simulink model "ar2_pos_123"  (R2019b)
settings: Solver=VariableStepAuto  StartTime=0.0  StopTime=10
libraries: simulink x3
settings Model: Creator=ah501846  LastModifiedBy=ah501846

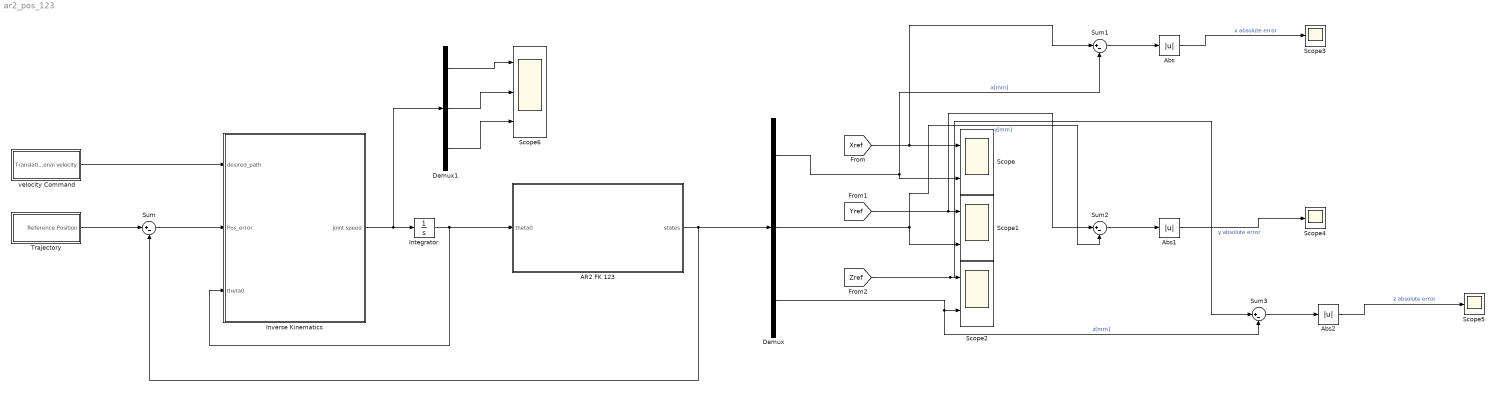
== system ar2_pos_123 ==
  AR2 FK 123 : MATLAB Function  TreatAsAtomicUnit=on
  Abs : Abs
  Abs1 : Abs
  Abs2 : Abs
  Demux : Demux  Outputs=3
  Demux1 : Demux  Outputs=3
  Integrator : Integrator  InitialCondition=[40 50 130 ]'*pi/180
  Inverse Kinematics : Subsystem
  Scope : Scope  NumInputPorts=2
  Scope1 : Scope  NumInputPorts=2
  Scope2 : Scope  NumInputPorts=2
  Scope3 : Scope
  Scope4 : Scope
  Scope5 : Scope
  Scope6 : Scope  NumInputPorts=3
  Sum{,1..3} (4 alike) : Sum  Inputs=|+-
  "Trajectory " : Subsystem
  velocity Command : Subsystem
  wires:
  "Trajectory "/1(Reference Position) -> Sum/1
  Sum/1 -> Inverse Kinematics/2(Pos_error)
  Inverse Kinematics/1(joint speed) -> Demux1/1, Integrator/1
  velocity Command/1(Translational velocity) -> Inverse Kinematics/1(desired_path)
  Integrator/1 -> AR2 FK 123/1(theta0), Inverse Kinematics/3(theta0)
  AR2 FK 123/1(states) -> Sum/2, Demux/1
  Abs1/1 -> Scope4/1  "y absolute error"
  Sum2/1 -> Abs1/1
  [Zref] -> Sum3/1, Scope2/1
  Sum1/1 -> Abs/1
  Abs/1 -> Scope3/1  "x absolute error"
  Demux/2 -> Scope1/2, Sum2/2  "y[mm]"
  Demux/3 -> Sum3/2, Scope2/2  "z[mm]"
  [Yref] -> Sum2/1, Scope1/1
  [Xref] -> Sum1/1, Scope/1
  Demux/1 -> Scope/2, Sum1/2  "x[mm]"
  Abs2/1 -> Scope5/1  "z absolute error"
  Sum3/1 -> Abs2/1
  Demux1/3 -> Scope6/3
  Demux1/2 -> Scope6/2
  Demux1/1 -> Scope6/1

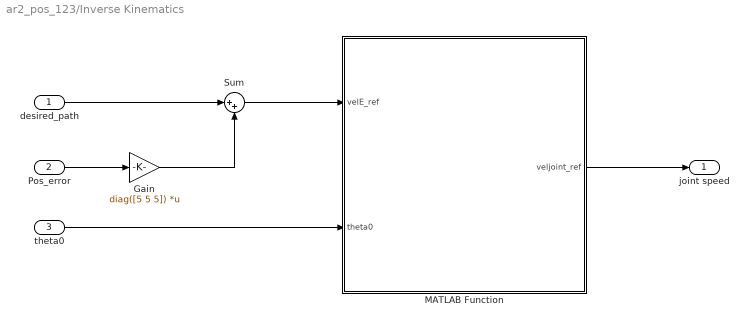
== system ar2_pos_123/Inverse Kinematics ==
  desired_path : Inport
  Pos_error : Inport  Port=2
  theta0 : Inport  Port=3
  Gain : Gain  Gain=diag([5 5 5])  Multiplication=Matrix(K*u)
  MATLAB Function : MATLAB Function  TreatAsAtomicUnit=on
  Sum : Sum  Inputs=|++
  joint speed : Outport  VectorParamsAs1DForOutWhenUnconnected=off
  wires:
  MATLAB Function/1(veljoint_ref) -> joint speed/1
  theta0/1 -> MATLAB Function/2(theta0)
  desired_path/1 -> Sum/1
  Sum/1 -> MATLAB Function/1(velE_ref)
  Pos_error/1 -> Gain/1
  Gain/1 -> Sum/2

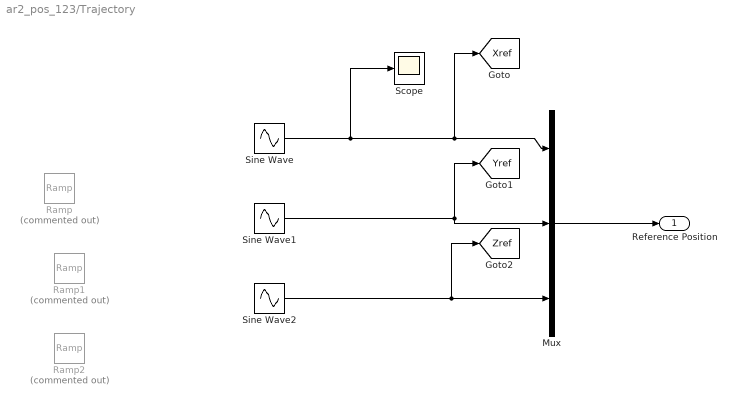
== system ar2_pos_123/Trajectory  ==
  Mux : Mux  Inputs=3
  Ramp : simulink/Sources/Ramp  Commented=on  slope=1  start=0  InitialOutput=195
  Ramp1 : simulink/Sources/Ramp  Commented=on  slope=1  start=0  InitialOutput=165
  Ramp2 : simulink/Sources/Ramp  Commented=on  slope=1  start=0  InitialOutput=-52
  Scope : Scope
  Sine Wave : Sin  Amplitude=50  Bias=195  SampleTime=0
  Sine Wave1 : Sin  Amplitude=50  Bias=165  SampleTime=0
  Sine Wave2 : Sin  Amplitude=50  Bias=-52  SampleTime=0
  Reference Position : Outport  VectorParamsAs1DForOutWhenUnconnected=off
  tag scope: Xref=global, Yref=global, Zref=global
  wires:
  Mux/1 -> Reference Position/1
  Sine Wave/1 -> Scope/1, Mux/1, [Xref]
  Sine Wave1/1 -> [Yref], Mux/2
  Sine Wave2/1 -> Mux/3, [Zref]

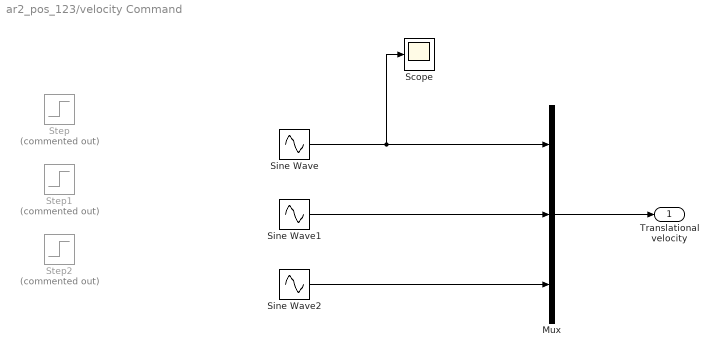
== system ar2_pos_123/velocity Command ==
  Mux : Mux  Inputs=3
  Scope : Scope
  Sine Wave : Sin  Amplitude=50  Phase=pi/2  SampleTime=0
  Sine Wave1 : Sin  Amplitude=50  Phase=pi/2  SampleTime=0
  Sine Wave2 : Sin  Amplitude=50  Phase=pi/2  SampleTime=0
  Step : Step  Commented=on  Time=10  SampleTime=0
  Step1 : Step  Commented=on  Time=10  SampleTime=0
  Step2 : Step  Commented=on  Time=10  SampleTime=0
  Translational velocity : Outport  VectorParamsAs1DForOutWhenUnconnected=off
  wires:
  Mux/1 -> Translational velocity/1
  Sine Wave/1 -> Scope/1, Mux/1
  Sine Wave1/1 -> Mux/2
  Sine Wave2/1 -> Mux/3

== matlab function ar2_pos_123/AR2 FK 123 ==
  data: states output; theta0 input
% function to calculate analytical Jacobian 
function states = manipFK(theta0)
%% Inputs
theta1 = theta0(1);
theta2 = theta0(2);
theta3 = theta0(3);
%% DH parameters
d1 = 169.77;    a1 = 64.2;  alpha1 = -90*pi/180;    
d2 = 0;         a2 = 305;   alpha2 = 0;             
d3 = 0;         a3 = 0;     alpha3 = 90*pi/180;     
d4 = -222.63;   a4 = 0;     alpha4 = -90*pi/180;    
d5 = 0;         a5 = 0;     alpha5 = 90*pi/180;     
d6 = -36.25;    a6 = 0;     alpha6 = 0;             
%% Direct Forward Kinematics
DH1 = [cos(theta1) -sin(theta1)*cos(alpha1) sin(theta1)*sin(alpha1) a1*cos(theta1);
       sin(theta1) cos(theta1)*cos(alpha1) -cos(theta1)*sin(alpha1) a1*sin(theta1); 
        0           sin(alpha1)             cos(alpha1)             d1;
        0 0 0 1];
DH2 = [cos(theta2) -sin(theta2)*cos(alpha2) sin(theta2)*sin(alpha2)     a2*cos(theta2);
        sin(theta2) cos(theta2)*cos(alpha2) -cos(theta2)*sin(alpha2)    a2*sin(theta2);
        0           sin(alpha2)             cos(alpha2)                 d2;
    0 0 0 1];
DH3 = [cos(theta3) -sin(theta3)*cos(alpha3) sin(theta3)*sin(alpha3) a3*cos(theta3);
    sin(theta3) cos(theta3)*cos(alpha3) -cos(theta3)*sin(alpha3)    a3*sin(theta3);
    0 sin(alpha3) cos(alpha3)                                       d3;
    0 0 0 1];
%% Homogeneous Transformation Matrix of the end effector to the base
HT3 = DH1*DH2*DH3;
%% Position
l1 = d1;
l2 = a2;
l3 = d4;
x = cos(theta1)*(l2*cos(theta2) + l3*sin(theta2+theta3));
y = sin(theta1) * (l2*cos(theta2) + l3*sin(theta2+theta3) );
z = l1 - l3*cos(theta2 + theta3) + l2*sin(theta2);
%% Outputs
states =  [x y z]';

== matlab function ar2_pos_123/Inverse Kinematics/MATLAB Function ==
  data: velE_ref input; veljoint_ref output; theta0 input
function veljoint_ref = trajectoryIK(velE_ref,theta0)

d1 = 169.77;    a1 = 64.2;  alpha1 = -90*pi/180;
d2 = 0;         a2 = 305;   alpha2 = 0;
d3 = 0;         a3 = 0;     alpha3 = 90*pi/180;
d4 = -222.63;   a4 = 0;     alpha4 = -90*pi/180;
d5 = 0;         a5 = 0;     alpha5 = 90*pi/180;
d6 = -36.25;    a6 = 0;     alpha6 = 0;

theta1 = theta0(1);
theta2 = theta0(2);
theta3 = theta0(3);
theta23 = theta2 + theta3;

cth1 = cos(theta1);
cth2 = cos(theta2);
cth3 = cos(theta3);
cth23 = cos(theta23);
sth1 = sin(theta1);
sth2 = sin(theta2);
sth3 = sin(theta3);
sth23 = sin(theta23);

cal1 = cos(alpha1);
cal2 = cos(alpha2);
cal3 = cos(alpha3);

sal1 = sin(alpha1);
sal2 = sin(alpha2);
sal3 = sin(alpha3);


% Jv3 = ([[d3*(cal2*sal1*cth1 - sal2*sth1*sth2 + cal1*sal2*cth1*cth2) - a1*sth1 + d2*sal1*cth1 + a3*sth3*(sal1*sal2*cth1 + cal2*sth1*sth2 - cal1*cal2*cth1*cth2) - a2*cth2*sth1 - a3*cth3*(cth2*sth1 + cal1*cth1*sth2) - a2*cal1*cth1*sth2, d3*(sal2*cth1*cth2 - cal1*sal2*sth1*sth2) - a2*cth1*sth2 - a3*sth3*(cal2*cth1*cth2 - cal1*cal2*sth1*sth2) - a3*cth3*(cth1*sth2 + cal1*cth2*sth1) - a2*cal1*cth2*sth1, - a3*sth3*(cth1*cth2 - cal1*sth1*sth2) - a3*cth3*(cal2*cth1*sth2 - sal1*sal2*sth1 + cal1*cal2*cth2*sth1)]; 
% [a1*cth1 + d3*(cal2*sal1*sth1 + sal2*cth1*sth2 + cal1*sal2*cth2*sth1) + a2*cth1*cth2 + d2*sal1*sth1 - a3*sth3*(cal2*cth1*sth2 - sal1*sal2*sth1 + cal1*cal2*cth2*sth1) + a3*cth3*(cth1*cth2 - cal1*sth1*sth2) - a2*cal1*sth1*sth2, d3*(sal2*cth2*sth1 + cal1*sal2*cth1*sth2) - a2*sth1*sth2 - a3*sth3*(cal2*cth2*sth1 + cal1*cal2*cth1*sth2) - a3*cth3*(sth1*sth2 - cal1*cth1*cth2) + a2*cal1*cth1*cth2, - a3*sth3*(cth2*sth1 + cal1*cth1*sth2) - a3*cth3*(sal1*sal2*cth1 + cal2*sth1*sth2 - cal1*cal2*cth1*cth2)]; 
% [0, a2*sal1*cth2 + a3*sal1*cth2*cth3 + d3*sal1*sal2*sth2 - a3*cal2*sal1*sth2*sth3, a3*cth3*(cal1*sal2 + cal2*sal1*cth2) - a3*sal1*sth2*sth3]]); 


l1 = d1;
l2 = a2;
l3 = d4;

Jv3 = [-(l3*sth23 + l2*cth2)*sth1    (l3*cth23 - l2*sth2)*cth1   l3*cth23*cth1;
       (l3*sth23 + l2*cth2)*cth1     (l3*cth23 - l2*sth2)*sth1  l3*cth23*sth1;
       0                             l3*sth23 + l2*cth2         l3*sth23];


% NOT WORKING
% Jv3 = [-(sth1*sth23*l3 + l2*cth2*sth1),   cth1*(-l2*sth2 + l3*cth23),     l3*cth1*sth23;      
%        l3*cth1*sth23 + l2*cth1*cth2,    sth1*(-l2*sth2 + l3*cth23),     l3*sth1*sth23;
%        0,                               l2*cth2 + l3*sth23,             -l3*cth23];



veljoint_ref = pinv(Jv3)*velE_ref;
